simulink model "FiltroV0"  (R2024b)
settings: Solver=VariableStepAuto  StartTime=0.0  StopTime=10.0  RelTol=1e-3
libraries: dspfdesign x5, dspvision x1
settings Model: Creator=fredy  LastModifiedBy=fredy

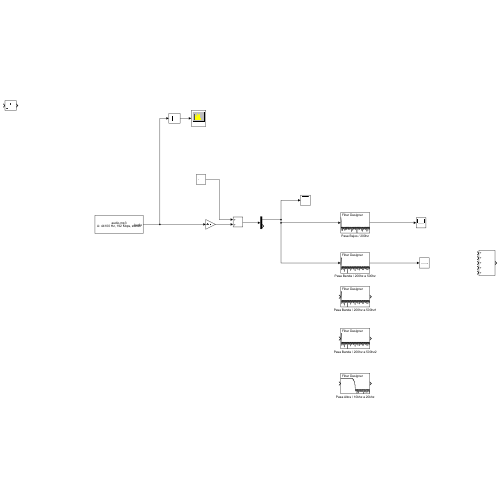
[thumbnail: Simulink's stored preview of the top-level diagram]
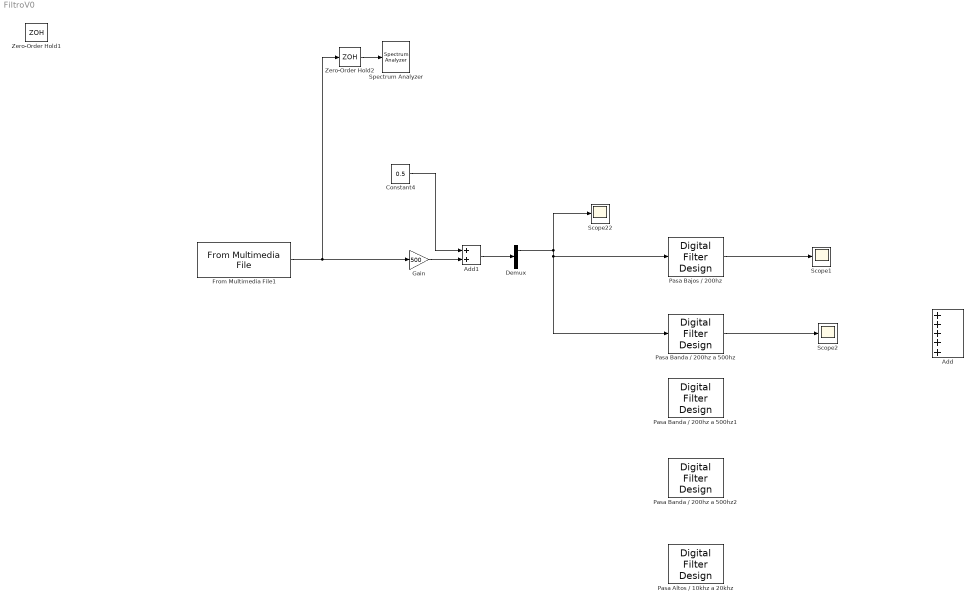
== system FiltroV0 ==
  Add : Sum  Inputs=+++++
  Add1 : Sum
  Constant4 : Constant  Value=0.5
  Demux : Demux  Outputs=2
  From Multimedia File1 : dspvision/From Multimedia File  inputFilename=D:\Datos Fredy\Programacion\Matlab\Filtros\audio.mp3  readRange=[1 Inf]  loop=on  numPlays=inf  outputStreams=Audio only  videoDataType=single  audioDataType=single  inheritSampleTime=on  userDefinedSampleTime=1/30  noAudioOutput=off  isIntensityVideo=off  fourcc=RGB  colorVideoFormat=Separate color signals  outputEOF=off  dataOrg=Column-major  audioFrameSize=1  computeAudioFrameSize=off  outSamplingMode=Sample based
      settings: LibrarySourceBlock=audiosources/From Multimedia File
  Gain : Gain  Gain=500
  Pasa Altos / 10khz a 20khz : dspfdesign/Digital Filter Design  mwdsp_browser_bugfix_var=off
  Pasa Bajos / 200hz : dspfdesign/Digital Filter Design  mwdsp_browser_bugfix_var=off
  Pasa Banda / 200hz a 500hz : dspfdesign/Digital Filter Design  mwdsp_browser_bugfix_var=off
  Pasa Banda / 200hz a 500hz1 : dspfdesign/Digital Filter Design  mwdsp_browser_bugfix_var=off
  Pasa Banda / 200hz a 500hz2 : dspfdesign/Digital Filter Design  mwdsp_browser_bugfix_var=off
  Scope1 : Scope
  Scope2 : Scope
  Scope22 : Scope
  Spectrum Analyzer : SpectrumAnalyzer  WindowPosition=[120.000000,629.000000,1132.000000,626.000000,]  ScopeFrameLocation=window  SampleRate=44.1e3  PlotAsTwoSidedSpectrum=off  FrequencyScale=Log  WindowInvariantSamplesPerUpdate=on  FrequencySpan=Start and stop frequencies  StartFrequency=20  YLimits=[-60.82132392,9.3898003]  SelectedToolstripTab=spectrumAnalyzerToolstrip.estimationTab
  Zero-Order Hold1 : ZeroOrderHold  SampleTime=0.0001
  Zero-Order Hold2 : ZeroOrderHold  SampleTime=0.0001
  wires:
  Add1/1 -> Demux/1
  Constant4/1 -> Add1/1
  Gain/1 -> Add1/2
  From Multimedia File1/1 -> Zero-Order Hold2/1, Gain/1
  Demux/1 -> Pasa Banda / 200hz a 500hz/1, Pasa Bajos / 200hz/1, Scope22/1
  Zero-Order Hold2/1 -> Spectrum Analyzer/1
  Pasa Bajos / 200hz/1 -> Scope1/1
  Pasa Banda / 200hz a 500hz/1 -> Scope2/1
